simulink model "Mul"  (R2022a)
settings: Solver=FixedStepDiscrete  StartTime=0.0  StopTime=10.0  RelTol=1e-3
settings Model: DataTypeOverride=Off  Creator=Ruwinda Nanayakkara  LastModifiedBy=Ruwinda Nanayakkara
settings SolverCC: AlgebraicLoopSolver=TrustRegion
settings DataIOCC: SaveOutput=off  SaveTime=off
settings OptimizationCC: BlockReduction=off  ConditionallyExecuteInputs=off  DefaultParameterBehavior=Inlined
settings DebuggingCC: AlgebraicLoopMsg=error  SingleTaskRateTransMsg=error  UnconnectedInputMsg=warning  UnconnectedOutputMsg=warning  UnconnectedLineMsg=warning  StrictBusMsg=ErrorOnBusTreatedAsVector  SFMachineParentedDataDiag=warning  ArithmeticOperatorsInVariantConditions=warning
settings HardwareCC: ProdBitPerPointer=32  ProdBitPerSizeT=32  ProdBitPerPtrDiffT=32  ProdLargestAtomicFloat=None  ProdIntDivRoundTo=Undefined  ProdEndianess=Unspecified  ProdWordSize=32  ProdHWDeviceType=ASIC/FPGA->ASIC/FPGA  ProdEqTarget=off
settings SFSimCC: SimUseLocalCustomCode=off  CustomCodeUndefinedFunction=UseInterfaceOnly
settings RTWCC: RTWUseLocalCustomCode=off
settings CodeAppCC: StateflowObjectComments=on
settings GRTTargetCC: TargetLangStandard=C89/C90 (ANSI)

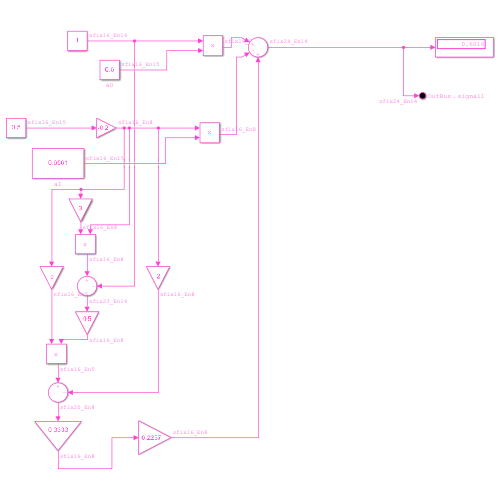
[thumbnail: Simulink's stored preview of the top-level diagram]
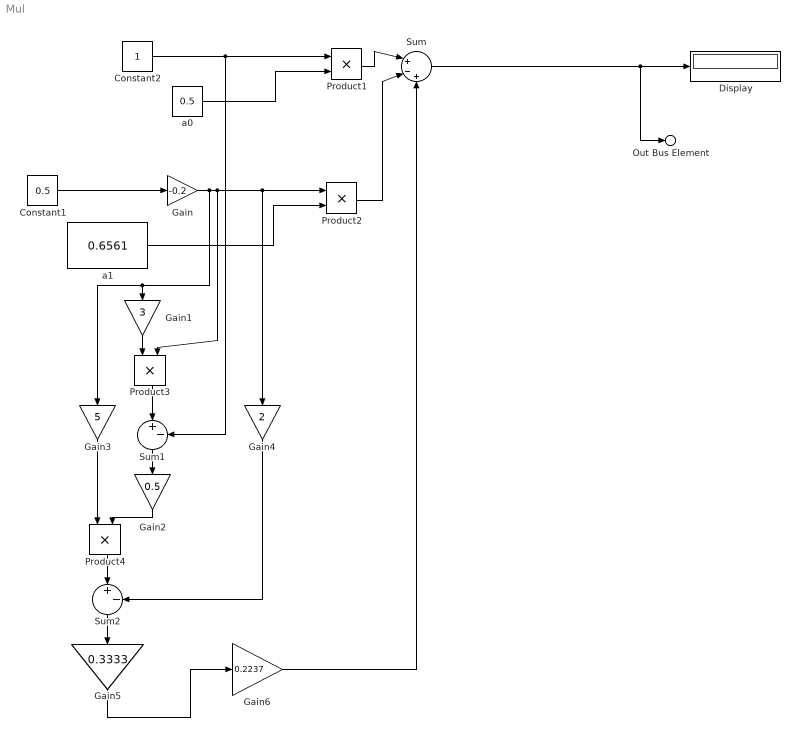
== system Mul ==
  Constant1 : Constant  Value=0.5  OutDataTypeStr=fixdt(1,16)
  Constant2 : Constant  OutDataTypeStr=fixdt(1,16)
  Display : Display
  Gain : Gain  Gain=-0.2  OutDataTypeStr=fixdt(1,16,8)
  Gain1 : Gain  Gain=3  OutDataTypeStr=fixdt(1,16,8)
  Gain2 : Gain  Gain=0.5  OutDataTypeStr=fixdt(1,16,8)
  Gain3 : Gain  Gain=5  OutDataTypeStr=fixdt(1,16,5)
  Gain4 : Gain  Gain=2  OutDataTypeStr=fixdt(1,16,8)
  Gain5 : Gain  Gain=0.3333  OutDataTypeStr=fixdt(1,16,8)
  Gain6 : Gain  Gain=0.2237  OutDataTypeStr=fixdt(1,16,8)
  Product{1..4} (4 alike) : Product  OutDataTypeStr=Inherit: Same as first input
  Sum : Sum  Inputs=|+-+
  Sum1 : Sum  Inputs=|+-
  Sum2 : Sum  Inputs=|+-
  a0 : Constant  Value=0.5  OutDataTypeStr=fixdt(1,16)
  a1 : Constant  Value=0.6561  VectorParams1D=off  OutDataTypeStr=fixdt(1,16)  LockScale=on
  Out Bus Element : Outport  VectorParamsAs1DForOutWhenUnconnected=off  PortName=OutBus  Element=signal1
  wires:
  Constant2/1 -> Product1/1, Sum1/2
  a0/1 -> Product1/2
  a1/1 -> Product2/2
  Product1/1 -> Sum/1
  Product2/1 -> Sum/2
  Sum/1 -> Display/1, Out Bus Element/1
  Constant1/1 -> Gain/1
  Gain/1 -> Gain3/1, Gain1/1, Product3/2, Product2/1, Gain4/1
  Gain1/1 -> Product3/1
  Product3/1 -> Sum1/1
  Sum1/1 -> Gain2/1
  Gain3/1 -> Product4/1
  Gain2/1 -> Product4/2
  Product4/1 -> Sum2/1
  Gain4/1 -> Sum2/2
  Sum2/1 -> Gain5/1
  Gain5/1 -> Gain6/1
  Gain6/1 -> Sum/3
